simulink model "output_mux_core"  (R2013a)
settings: Solver=ode45  StartTime=0.0  StopTime=10.0  RelTol=1e-3
libraries: xbsIndex_r4 x496, casper_library_misc x1
(part 2 of 2)

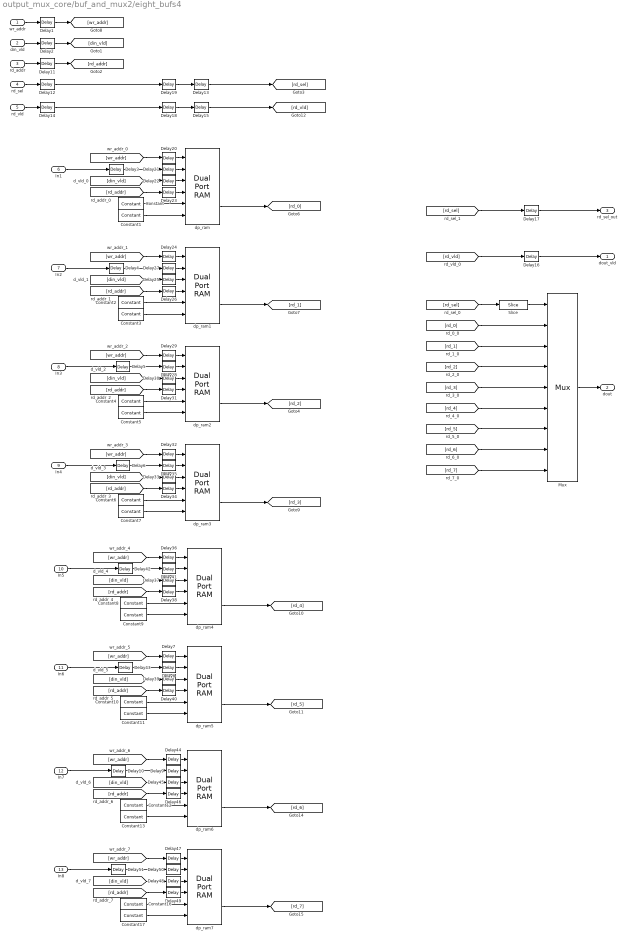
== system output_mux_core/buf_and_mux2/eight_bufs4 ==
  wr_addr : Inport
  din_vld : Inport  Port=2
  rd_addr : Inport  Port=3
  rd_sel : Inport  Port=4
  rd_vld : Inport  Port=5
  In1 : Inport  Port=6
  In2 : Inport  Port=7
  In3 : Inport  Port=8
  In4 : Inport  Port=9
  In5 : Inport  Port=10
  In6 : Inport  Port=11
  In7 : Inport  Port=12
  In8 : Inport  Port=13
  Constant{,2,4,6,8,10,12,16} (8 alike) : xbsIndex_r4/Constant  const=0  gui_display_data_type=Fixed-point  arith_type=Unsigned  n_bits=64  bin_pt=0  preci_type=Single  exp_width=8  frac_width=24  explicit_period=on  period=1  equ=P=C  opselect=C  inp2=PCIN>>17  opr=+  inp1=P  carry=CIN  dbl_ovrd=off  block_type=constant
  Constant{1,3,5,7,9,11,13,17} (8 alike) : xbsIndex_r4/Constant  const=0  gui_display_data_type=Boolean  arith_type=Boolean  n_bits=64  bin_pt=0  preci_type=Single  exp_width=8  frac_width=24  explicit_period=on  period=1  equ=P=C  opselect=C  inp2=PCIN>>17  opr=+  inp1=P  carry=CIN  dbl_ovrd=off  block_type=constant
  Delay{1..2,7,11..12,14,20,22..26,29..34,36..40,44..49} (29 alike) : xbsIndex_r4/Delay  rst=off  infoeditControl=Selection of Reset will increase slice count due to use of real FFs and instead of SRLs  en=off  latency=1  dbl_ovrd=off  reg_retiming=off  block_type=delay
  Delay{3..6,8..10,18..19,21,27..28,35,41..43,50..51} (18 alike) : xbsIndex_r4/Delay  rst=off  infoeditControl=Selection of Reset will increase slice count due to use of real FFs and instead of SRLs  en=off  latency=1  dbl_ovrd=off  reg_retiming=on  block_type=delay
  Delay13 : xbsIndex_r4/Delay  rst=off  infoeditControl=Selection of Reset will increase slice count due to use of real FFs and instead of SRLs  en=off  latency=3  dbl_ovrd=off  reg_retiming=on  block_type=delay
  Delay15 : xbsIndex_r4/Delay  rst=off  infoeditControl=Selection of Reset will increase slice count due to use of real FFs and instead of SRLs  en=off  latency=3  dbl_ovrd=off  reg_retiming=on  block_type=delay
  Delay16 : xbsIndex_r4/Delay  rst=off  infoeditControl=Selection of Reset will increase slice count due to use of real FFs and instead of SRLs  en=off  latency=2  dbl_ovrd=off  reg_retiming=off  block_type=delay
  Delay17 : xbsIndex_r4/Delay  rst=off  infoeditControl=Selection of Reset will increase slice count due to use of real FFs and instead of SRLs  en=off  latency=2  dbl_ovrd=off  reg_retiming=off  block_type=delay
  Mux : xbsIndex_r4/Mux  inputs=8  en=off  latency=2  precision=Full  arith_type=Unsigned  n_bits=16  bin_pt=14  quantization=Truncate  overflow=Wrap  dbl_ovrd=off  block_type=mux
  Slice : xbsIndex_r4/Slice  nbits=3  boolean_output=off  mode=Lower Bit Location + Width  bit1=0  base1=MSB of Input  bit0=0  base0=LSB of Input  dbl_ovrd=off  block_type=slice
  dp_ram{,1..7} (8 alike) : xbsIndex_r4/Dual Port RAM  depth=2^bram_depth  initVector=sin(pi*(0:15)/16)  distributed_mem=Block RAM  init_a=0  init_b=0  rst_a=off  rst_b=off  en_a=off  en_b=off  latency=3  write_mode_A=Read After Write  write_mode_B=Read After Write  dbl_ovrd=off  optimize=Speed  block_type=dpram
  dout_vld : Outport
  dout : Outport  Port=2
  rd_sel_out : Outport  Port=3
  wires:
  Slice/1 -> Mux/1
  Delay17/1 -> rd_sel_out/1
  [rd_sel] -> Delay17/1
  Delay16/1 -> dout_vld/1
  [rd_vld] -> Delay16/1
  Delay14/1 -> Delay18/1
  Delay15/1 -> [rd_vld]
  rd_vld/1 -> Delay14/1
  Mux/1 -> dout/1
  [rd_1] -> Mux/3
  [rd_2] -> Mux/4
  [rd_0] -> Mux/2
  [rd_5] -> Mux/7
  [rd_4] -> Mux/6
  [rd_sel] -> Slice/1
  [rd_7] -> Mux/9
  [rd_6] -> Mux/8
  [rd_3] -> Mux/5
  dp_ram7/2 -> [rd_7]
  dp_ram6/2 -> [rd_6]
  dp_ram5/2 -> [rd_5]
  dp_ram4/2 -> [rd_4]
  dp_ram3/2 -> [rd_3]
  dp_ram2/2 -> [rd_2]
  dp_ram1/2 -> [rd_1]
  dp_ram/2 -> [rd_0]
  Delay13/1 -> [rd_sel]
  Delay12/1 -> Delay19/1
  rd_sel/1 -> Delay12/1
  Delay11/1 -> [rd_addr]
  rd_addr/1 -> Delay11/1
  Delay2/1 -> [din_vld]
  din_vld/1 -> Delay2/1
  Delay1/1 -> [wr_addr]
  wr_addr/1 -> Delay1/1
  Constant1/1 -> dp_ram/6
  [wr_addr] -> Delay44/1
  Constant17/1 -> dp_ram7/6
  [wr_addr] -> Delay7/1
  [din_vld] -> Delay22/1
  [din_vld] -> Delay39/1
  Delay4/1 -> Delay27/1
  Delay51/1 -> Delay50/1
  [rd_addr] -> Delay46/1
  Constant7/1 -> dp_ram3/6
  In4/1 -> Delay6/1
  Constant11/1 -> dp_ram5/6
  Constant13/1 -> dp_ram6/6
  Delay42/1 -> Delay41/1
  [din_vld] -> Delay33/1
  Constant10/1 -> dp_ram5/5
  [rd_addr] -> Delay38/1
  Constant4/1 -> dp_ram2/5
  Constant12/1 -> dp_ram6/5
  Constant8/1 -> dp_ram4/5
  [din_vld] -> Delay30/1
  Delay43/1 -> Delay8/1
  [din_vld] -> Delay48/1
  [din_vld] -> Delay37/1
  [rd_addr] -> Delay40/1
  In1/1 -> Delay3/1
  [rd_addr] -> Delay34/1
  Delay10/1 -> Delay9/1
  [rd_addr] -> Delay31/1
  Delay5/1 -> Delay28/1
  [wr_addr] -> Delay47/1
  Constant16/1 -> dp_ram7/5
  In6/1 -> Delay43/1
  Constant6/1 -> dp_ram3/5
  Constant9/1 -> dp_ram4/6
  In3/1 -> Delay5/1
  In8/1 -> Delay51/1
  [wr_addr] -> Delay36/1
  [wr_addr] -> Delay29/1
  In7/1 -> Delay10/1
  Constant/1 -> dp_ram/5
  Constant5/1 -> dp_ram2/6
  [rd_addr] -> Delay49/1
  In5/1 -> Delay42/1
  [wr_addr] -> Delay32/1
  [wr_addr] -> Delay20/1
  [wr_addr] -> Delay24/1
  [rd_addr] -> Delay26/1
  In2/1 -> Delay4/1
  Constant2/1 -> dp_ram1/5
  Constant3/1 -> dp_ram1/6
  [din_vld] -> Delay25/1
  [din_vld] -> Delay45/1
  [rd_addr] -> Delay23/1
  Delay3/1 -> Delay21/1
  Delay18/1 -> Delay15/1
  Delay19/1 -> Delay13/1
  Delay20/1 -> dp_ram/1
  Delay21/1 -> dp_ram/2
  Delay22/1 -> dp_ram/3
  Delay23/1 -> dp_ram/4
  Delay24/1 -> dp_ram1/1
  Delay25/1 -> dp_ram1/3
  Delay26/1 -> dp_ram1/4
  Delay27/1 -> dp_ram1/2
  Delay28/1 -> dp_ram2/2
  Delay29/1 -> dp_ram2/1
  Delay30/1 -> dp_ram2/3
  Delay31/1 -> dp_ram2/4
  Delay32/1 -> dp_ram3/1
  Delay33/1 -> dp_ram3/3
  Delay34/1 -> dp_ram3/4
  Delay6/1 -> Delay35/1
  Delay35/1 -> dp_ram3/2
  Delay36/1 -> dp_ram4/1
  Delay37/1 -> dp_ram4/3
  Delay38/1 -> dp_ram4/4
  Delay7/1 -> dp_ram5/1
  Delay39/1 -> dp_ram5/3
  Delay40/1 -> dp_ram5/4
  Delay41/1 -> dp_ram4/2
  Delay8/1 -> dp_ram5/2
  Delay44/1 -> dp_ram6/1
  Delay45/1 -> dp_ram6/3
  Delay46/1 -> dp_ram6/4
  Delay47/1 -> dp_ram7/1
  Delay48/1 -> dp_ram7/3
  Delay49/1 -> dp_ram7/4
  Delay9/1 -> dp_ram6/2
  Delay50/1 -> dp_ram7/2
